simulink model "quarter_car_active"  (R2025a)
settings: Solver=ode45  StartTime=0.0  StopTime=5  RelTol=1e-4  AbsTol=1e-6
InitFcn:
  | quarter_car_recalc_callback
values from neighbouring files (symbols this model uses):
  Mc = 300    [quarter_car_init.m]    (also in quarter_car_recalc_callback.m = str2double(Mc_str))
  Mw = 50    [quarter_car_init.m]    (also in quarter_car_recalc_callback.m = str2double(Mw_str))
  step_amp = 0.05    [quarter_car_init.m]    (also in quarter_car_recalc_callback.m)
undefined symbols (not defined in the file or in its folder): A_pid_cl, A_sf_cl, B_pid_cl, B_sf_cl, C_pid_cl, C_sf_cl, D_pid_cl, D_sf_cl
settings Model: Creator=donghankim  LastModifiedBy=donghankim

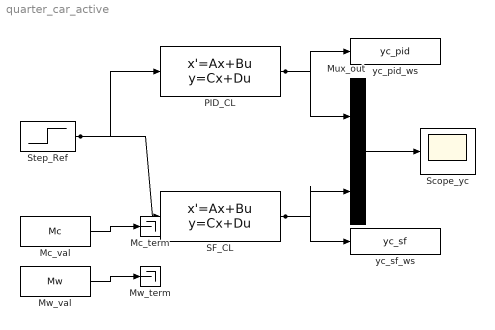
== system quarter_car_active ==
  Mc_term : Terminator
  Mc_val : Constant  Value=Mc
  Mux_out : Mux  Inputs=2
  Mw_term : Terminator
  Mw_val : Constant  Value=Mw
  PID_CL : StateSpace  A=A_pid_cl  B=B_pid_cl  C=C_pid_cl  D=D_pid_cl  InitialCondition=zeros(size(A_pid_cl,1),1)
  SF_CL : StateSpace  A=A_sf_cl  B=B_sf_cl  C=C_sf_cl  D=D_sf_cl  InitialCondition=zeros(size(A_sf_cl,1),1)
  Scope_yc : Scope
  Step_Ref : Step  Time=0  After=step_amp  SampleTime=0
  yc_pid_ws : ToWorkspace  VariableName=yc_pid  SampleTime=-1
  yc_sf_ws : ToWorkspace  VariableName=yc_sf  SampleTime=-1
  wires:
  Step_Ref/1 -> PID_CL/1, SF_CL/1
  PID_CL/1 -> Mux_out/1, yc_pid_ws/1
  SF_CL/1 -> Mux_out/2, yc_sf_ws/1
  Mux_out/1 -> Scope_yc/1
  Mc_val/1 -> Mc_term/1
  Mw_val/1 -> Mw_term/1
